simulink model "krstic_example_1p3_wnoise"  (Simulink 7.3)
settings: Solver=ode45  StartTime=0.0  StopTime=100  RelTol=1e-3
settings Model: Creator=sbrunton  LastModifiedBy=sbrunton
settings DataIOCC: LimitDataPoints=off

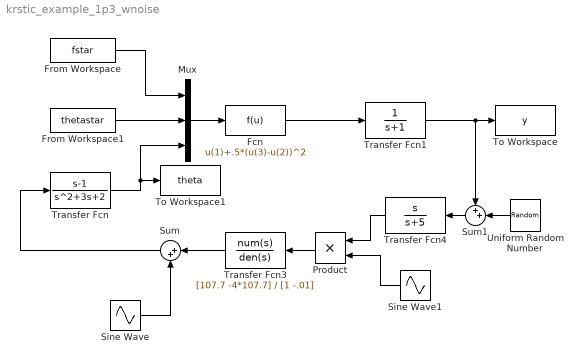
== system krstic_example_1p3_wnoise ==
  Fcn : Fcn  Expr=u(1)+.5*(u(3)-u(2))^2
  From Workspace : FromWorkspace  VariableName=fstar  SampleTime=0
  From Workspace1 : FromWorkspace  VariableName=thetastar  SampleTime=0
  Mux : Mux  Inputs=3
  Product : Product  OutDataType=fixdt(1, 16)  OutScaling=2^0  RndMeth=Zero
  Sine Wave : Sin  Amplitude=.05  Bias=0  Frequency=5  Phase=0  Samples=10  SampleTime=0  Offset=0
  Sine Wave1 : Sin  Amplitude=1  Bias=0  Frequency=5  Phase=.7955  Samples=10  SampleTime=0  Offset=0
  Sum : Sum  Inputs=|++  OutDataType=fixdt(1, 16)  OutScaling=2^0
  Sum1 : Sum  Inputs=++|  OutDataType=fixdt(1, 16)  OutScaling=2^0
  To Workspace : ToWorkspace  VariableName=y  SampleTime=-1  SaveFormat=Array
  To Workspace1 : ToWorkspace  VariableName=theta  SampleTime=-1  SaveFormat=Array
  Transfer Fcn : TransferFcn  Numerator=[1 -1]  Denominator=[1 3 2]
  Transfer Fcn1 : TransferFcn  Denominator=[1 1]
  Transfer Fcn3 : TransferFcn  Numerator=[107.7 -4*107.7]  Denominator=[1 -.01]
  Transfer Fcn4 : TransferFcn  Numerator=[1 0]  Denominator=[1 5]
  Uniform Random Number : UniformRandomNumber  Minimum=-.001  Maximum=.001  SampleTime=.001
  wires:
  Transfer Fcn1/1 -> To Workspace/1, Sum1/1
  Sum/1 -> Transfer Fcn/1
  From Workspace1/1 -> Mux/2
  From Workspace/1 -> Mux/1
  Transfer Fcn/1 -> Mux/3, To Workspace1/1
  Mux/1 -> Fcn/1
  Fcn/1 -> Transfer Fcn1/1
  Transfer Fcn4/1 -> Product/1
  Sine Wave1/1 -> Product/2
  Product/1 -> Transfer Fcn3/1
  Transfer Fcn3/1 -> Sum/1
  Sine Wave/1 -> Sum/2
  Sum1/1 -> Transfer Fcn4/1
  Uniform Random Number/1 -> Sum1/2
